simulink model "heaterWithRelay"  (R2020b)
settings: Solver=ode15s  StartTime=0  StopTime=7000  RelTol=1e-6
settings Model: Creator=avi  LastModifiedBy=avi
settings DataIOCC: Refine=4

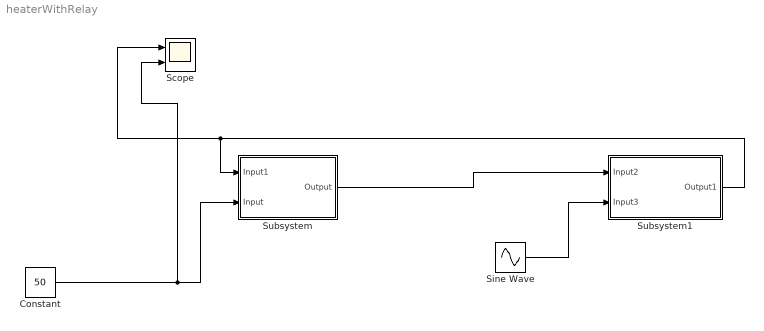
== system heaterWithRelay ==
  Constant : Constant  Value=50
  Scope : Scope  NumInputPorts=2
  Sine Wave : Sin  Amplitude=10  Bias=25  Frequency=0.00005  SampleTime=0
  Subsystem : Subsystem
  Subsystem1 : Subsystem
  wires:
  Constant/1 -> Scope/2, Subsystem/2(Input)
  Subsystem/1(Output) -> Subsystem1/1(Input2)
  Sine Wave/1 -> Subsystem1/2(Input3)
  Subsystem1/1(Output1) -> Scope/1, Subsystem/1(Input1)

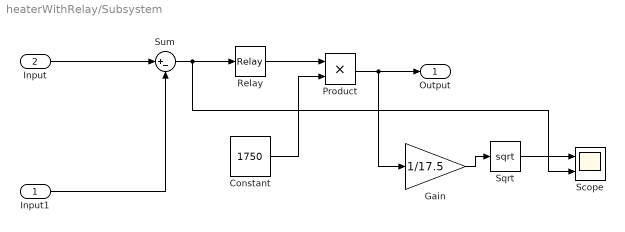
== system heaterWithRelay/Subsystem ==
  Input1 : Inport
  Input : Inport  Port=2
  Constant : Constant  Value=1750
  Gain : Gain  Gain=1/17.5
  Product : Product
  Relay : Relay  OnSwitchValue=3  OffSwitchValue=-3
  Scope : Scope  NumInputPorts=2
  Sqrt : Sqrt  SaturateOnIntegerOverflow=on
  Sum : Sum  Inputs=|+-
  Output : Outport
  wires:
  Input/1 -> Sum/1
  Constant/1 -> Product/2
  Input1/1 -> Sum/2
  Product/1 -> Output/1, Gain/1
  Relay/1 -> Product/1
  Gain/1 -> Sqrt/1
  Sum/1 -> Scope/2, Relay/1
  Sqrt/1 -> Scope/1

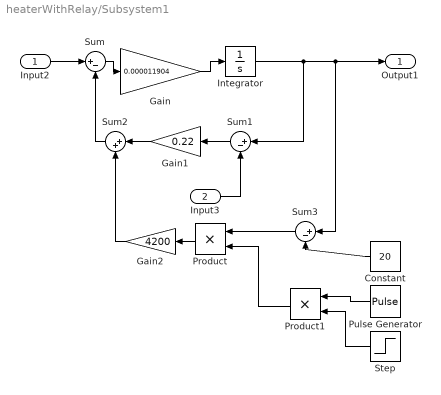
== system heaterWithRelay/Subsystem1 ==
  Input2 : Inport
  Input3 : Inport  Port=2
  Constant : Constant  Value=20
  Gain : Gain  Gain=0.000011904
  Gain1 : Gain  Gain=0.22
  Gain2 : Gain  Gain=4200
  Integrator : Integrator  InitialCondition=20
  Product : Product
  Product1 : Product
  Pulse Generator : DiscretePulseGenerator  PulseType=Time based  Amplitude=4.66/60  Period=300  PulseWidth=50  PhaseDelay=2500
  Step : Step  Time=2500  SampleTime=0
  Sum : Sum  Inputs=|+-
  Sum1 : Sum  Inputs=|+-
  Sum2 : Sum  Inputs=|++
  Sum3 : Sum  Inputs=|+-
  Output1 : Outport
  wires:
  Gain/1 -> Integrator/1
  Gain1/1 -> Sum2/1
  Sum/1 -> Gain/1
  Step/1 -> Product1/2
  Constant/1 -> Sum3/2
  Integrator/1 -> Sum1/1, Output1/1, Sum3/1
  Sum2/1 -> Sum/2
  Input3/1 -> Sum1/2
  Input2/1 -> Sum/1
  Sum1/1 -> Gain1/1
  Product/1 -> Gain2/1
  Gain2/1 -> Sum2/2
  Sum3/1 -> Product/1
  Product1/1 -> Product/2
  Pulse Generator/1 -> Product1/1
